simulink model "BH_base_simulink_formigas"  (R2021b)
settings: Solver=ode23tb  StartTime=0.0  StopTime=10  RelTol=1e-3
values from neighbouring files (symbols this model uses):
  a = 3.2    [BH_Otim_formigas.m]
  A1 = 1.2566e-3    (= 0.0012566)    [BH_Otim_formigas.m]
  A2 = 8.765e-4    (= 0.0008765)    [BH_Otim_formigas.m]
  be = 9000e5    (= 900000000)    [BH_Otim_formigas.m]
  f = 1500    [BH_Otim_formigas.m]
  g = 9.8    [BH_Otim_formigas.m]
  gama = 170    [BH_Otim_formigas.m]    (also in cost_func_bh.m = parameter(4))
  k1 = 11    [BH_Otim_formigas.m]    (also in cost_func_bh.m = parameter(5))
  k2 = 0.9    [BH_Otim_formigas.m]    (also in cost_func_bh.m = parameter(6))
  kc1 = 3.644e-12    [BH_Otim_formigas.m]
  kc2 = 4.376e-12    [BH_Otim_formigas.m]
  kq1 = 4.76e-4    (= 0.000476)    [BH_Otim_formigas.m]
  kq2 = 4.76e-4    (= 0.000476)    [BH_Otim_formigas.m]
  M = 84    [BH_Otim_formigas.m]    (also in cost_func_bh.m = M0 + exp(-5*s))
  M0 = 480    [BH_Otim_formigas.m]    (also in cost_func_bh.m = parameter(1))
  r0 = 0.62    [BH_Otim_formigas.m]    (also in cost_func_bh.m = parameter(3))
  V1 = VL1+(A1*xe0)    (= 0.0001330412)    [BH_Otim_formigas.m]
  V2 = VL2+A2*(L-xe0)    (= 0.000153427)    [BH_Otim_formigas.m]
libraries: simulink x1
settings Model: Creator=cof_2  LastModifiedBy=cof_2

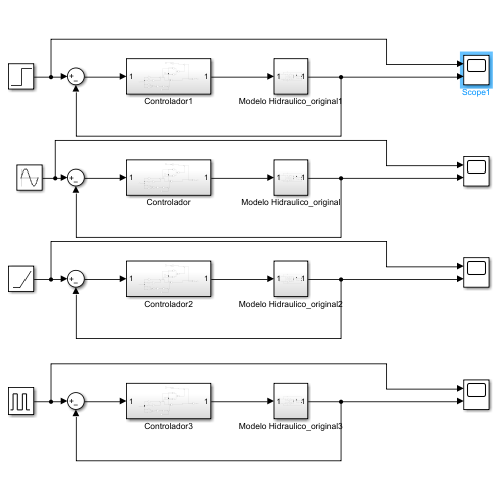
[thumbnail: Simulink's stored preview of the top-level diagram]
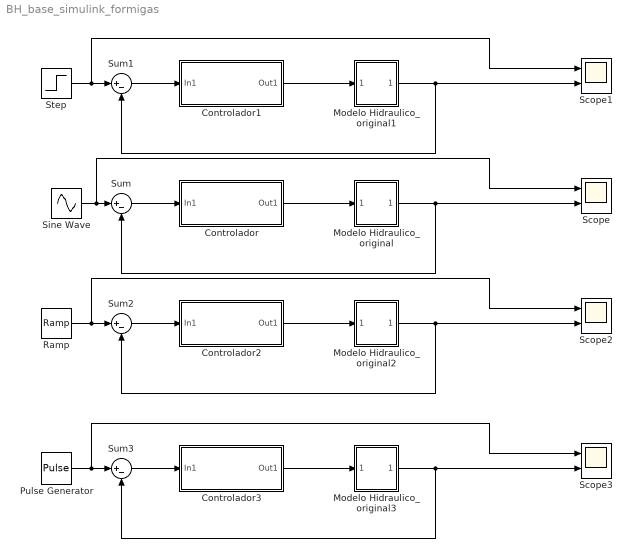
== system BH_base_simulink_formigas ==
  Controlador : Subsystem
  Controlador1 : Subsystem
  Controlador2 : Subsystem
  Controlador3 : Subsystem
  Modelo Hidraulico_original : Subsystem
  Modelo Hidraulico_original1 : Subsystem
  Modelo Hidraulico_original2 : Subsystem
  Modelo Hidraulico_original3 : Subsystem
  Pulse Generator : DiscretePulseGenerator  PulseType=Time based  Period=2.5  PulseWidth=5
  Ramp : simulink/Sources/Ramp  slope=1  start=0  InitialOutput=0
  Scope{,1..3} (4 alike) : Scope  NumInputPorts=2
  Sine Wave : Sin  SampleTime=0
  Step : Step  SampleTime=0
  Sum{,1..3} (4 alike) : Sum  Inputs=|+-
  wires:
  Controlador/1(Out1) -> Modelo Hidraulico_original/1(In1)
  Modelo Hidraulico_original/1(Out1) -> Sum/2, Scope/2
  Sum/1 -> Controlador/1(In1)
  Sine Wave/1 -> Scope/1, Sum/1
  Step/1 -> Sum1/1, Scope1/1
  Sum1/1 -> Controlador1/1(In1)
  Modelo Hidraulico_original1/1(Out1) -> Scope1/2, Sum1/2
  Controlador1/1(Out1) -> Modelo Hidraulico_original1/1(In1)
  Controlador2/1(Out1) -> Modelo Hidraulico_original2/1(In1)
  Modelo Hidraulico_original2/1(Out1) -> Sum2/2, Scope2/2
  Sum2/1 -> Controlador2/1(In1)
  Ramp/1 -> Scope2/1, Sum2/1
  Pulse Generator/1 -> Sum3/1, Scope3/1
  Sum3/1 -> Controlador3/1(In1)
  Modelo Hidraulico_original3/1(Out1) -> Scope3/2, Sum3/2
  Controlador3/1(Out1) -> Modelo Hidraulico_original3/1(In1)

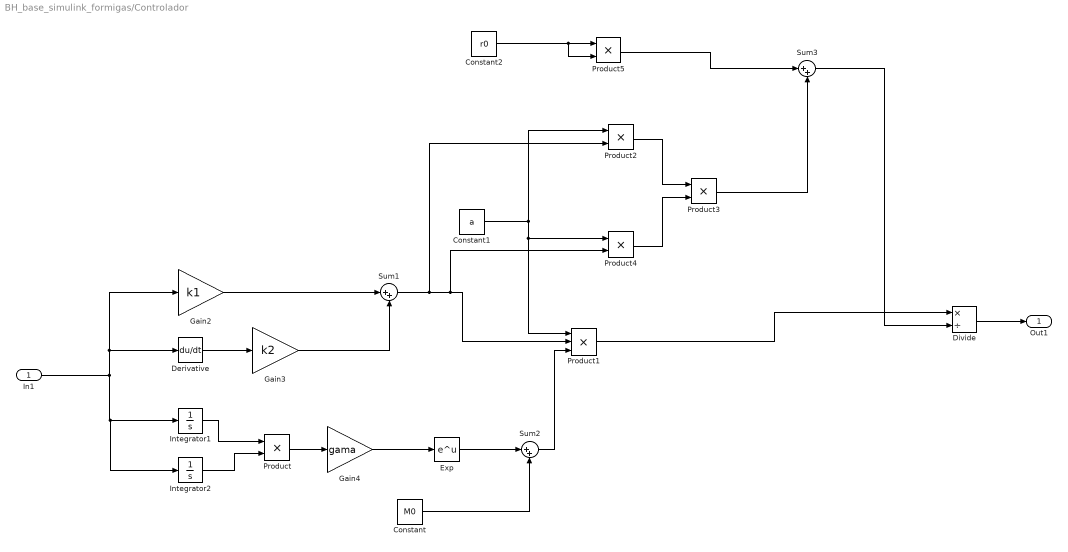
== system BH_base_simulink_formigas/Controlador ==
  In1 : Inport
  Constant : Constant  Value=M0
  Constant1 : Constant  Value=a
  Constant2 : Constant  Value=r0
  Derivative : Derivative
  Divide : Product  Inputs=*/
  Exp : Math  SaturateOnIntegerOverflow=on
  Gain2 : Gain  Gain=k1
  Gain3 : Gain  Gain=k2
  Gain4 : Gain  Gain=gama
  Integrator1 : Integrator
  Integrator2 : Integrator
  Product{,2..5} (5 alike) : Product
  Product1 : Product  Inputs=3
  Sum1 : Sum  Inputs=|++
  Sum2 : Sum  Inputs=|++
  Sum3 : Sum  Inputs=|++
  Out1 : Outport
  wires:
  In1/1 -> Gain2/1, Derivative/1, Integrator2/1, Integrator1/1
  Derivative/1 -> Gain3/1
  Integrator2/1 -> Product/2
  Integrator1/1 -> Product/1
  Product/1 -> Gain4/1
  Gain4/1 -> Exp/1
  Exp/1 -> Sum2/1
  Constant/1 -> Sum2/2
  Gain2/1 -> Sum1/1
  Gain3/1 -> Sum1/2
  Constant1/1 -> Product1/1, Product4/1, Product2/1
  Sum1/1 -> Product2/2, Product4/2, Product1/2
  Sum2/1 -> Product1/3
  Product2/1 -> Product3/1
  Product4/1 -> Product3/2
  Constant2/1 -> Product5/2, Product5/1
  Product5/1 -> Sum3/1
  Product3/1 -> Sum3/2
  Divide/1 -> Out1/1
  Product1/1 -> Divide/1
  Sum3/1 -> Divide/2

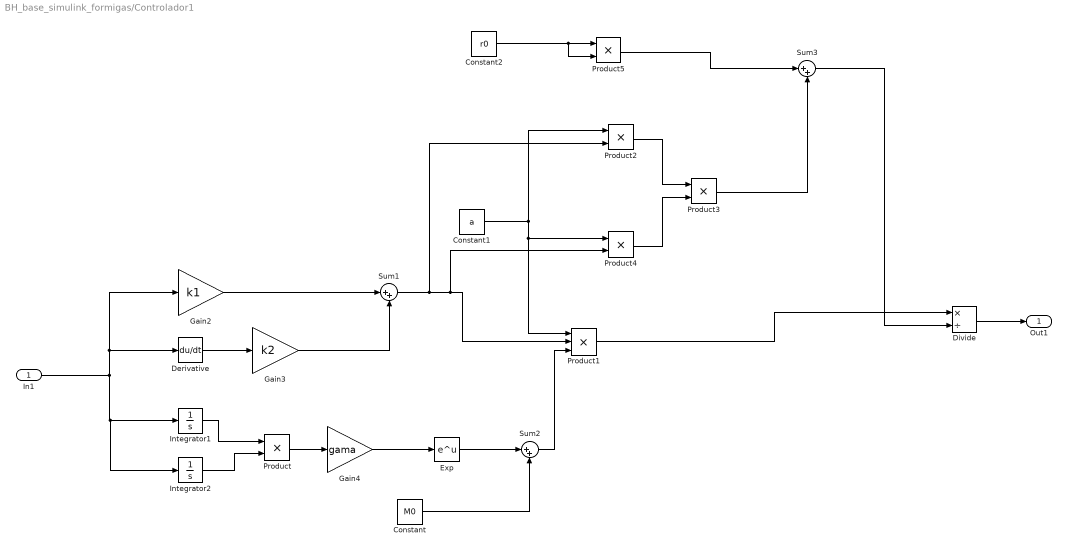
== system BH_base_simulink_formigas/Controlador1 ==
  In1 : Inport
  Constant : Constant  Value=M0
  Constant1 : Constant  Value=a
  Constant2 : Constant  Value=r0
  Derivative : Derivative
  Divide : Product  Inputs=*/
  Exp : Math  SaturateOnIntegerOverflow=on
  Gain2 : Gain  Gain=k1
  Gain3 : Gain  Gain=k2
  Gain4 : Gain  Gain=gama
  Integrator1 : Integrator
  Integrator2 : Integrator
  Product{,2..5} (5 alike) : Product
  Product1 : Product  Inputs=3
  Sum1 : Sum  Inputs=|++
  Sum2 : Sum  Inputs=|++
  Sum3 : Sum  Inputs=|++
  Out1 : Outport
  wires:
  Sum3/1 -> Divide/2
  Product1/1 -> Divide/1
  Divide/1 -> Out1/1
  Product3/1 -> Sum3/2
  Product5/1 -> Sum3/1
  Constant2/1 -> Product5/1, Product5/2
  Product4/1 -> Product3/2
  Product2/1 -> Product3/1
  Sum2/1 -> Product1/3
  Sum1/1 -> Product1/2, Product4/2, Product2/2
  Constant1/1 -> Product2/1, Product4/1, Product1/1
  Gain3/1 -> Sum1/2
  Gain2/1 -> Sum1/1
  Constant/1 -> Sum2/2
  Exp/1 -> Sum2/1
  Gain4/1 -> Exp/1
  Product/1 -> Gain4/1
  Integrator1/1 -> Product/1
  Integrator2/1 -> Product/2
  Derivative/1 -> Gain3/1
  In1/1 -> Integrator1/1, Integrator2/1, Derivative/1, Gain2/1

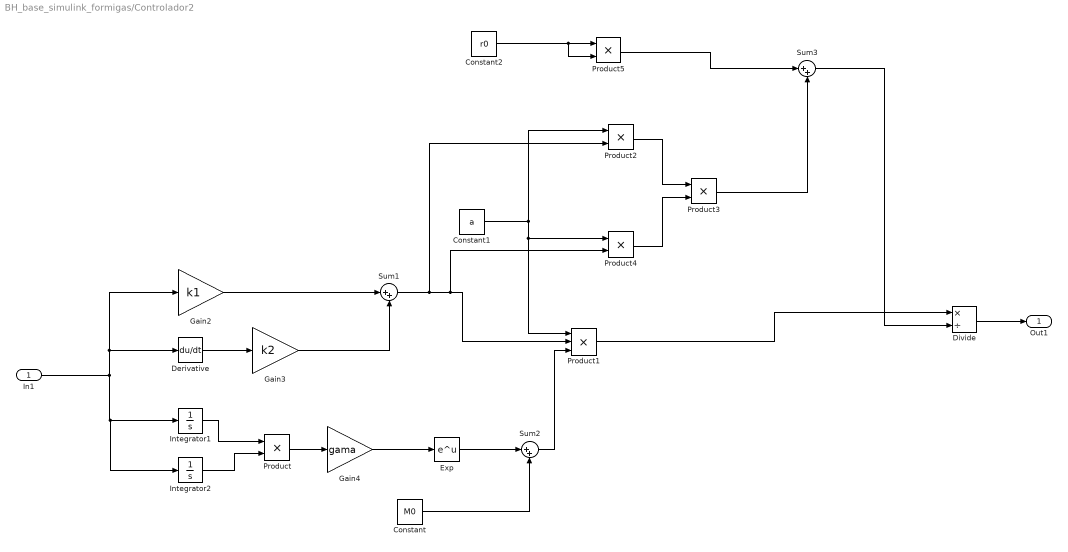
== system BH_base_simulink_formigas/Controlador2 ==
  In1 : Inport
  Constant : Constant  Value=M0
  Constant1 : Constant  Value=a
  Constant2 : Constant  Value=r0
  Derivative : Derivative
  Divide : Product  Inputs=*/
  Exp : Math  SaturateOnIntegerOverflow=on
  Gain2 : Gain  Gain=k1
  Gain3 : Gain  Gain=k2
  Gain4 : Gain  Gain=gama
  Integrator1 : Integrator
  Integrator2 : Integrator
  Product{,2..5} (5 alike) : Product
  Product1 : Product  Inputs=3
  Sum1 : Sum  Inputs=|++
  Sum2 : Sum  Inputs=|++
  Sum3 : Sum  Inputs=|++
  Out1 : Outport
  wires:
  In1/1 -> Gain2/1, Derivative/1, Integrator2/1, Integrator1/1
  Derivative/1 -> Gain3/1
  Integrator2/1 -> Product/2
  Integrator1/1 -> Product/1
  Product/1 -> Gain4/1
  Gain4/1 -> Exp/1
  Exp/1 -> Sum2/1
  Constant/1 -> Sum2/2
  Gain2/1 -> Sum1/1
  Gain3/1 -> Sum1/2
  Constant1/1 -> Product1/1, Product4/1, Product2/1
  Sum1/1 -> Product2/2, Product4/2, Product1/2
  Sum2/1 -> Product1/3
  Product2/1 -> Product3/1
  Product4/1 -> Product3/2
  Constant2/1 -> Product5/2, Product5/1
  Product5/1 -> Sum3/1
  Product3/1 -> Sum3/2
  Divide/1 -> Out1/1
  Product1/1 -> Divide/1
  Sum3/1 -> Divide/2

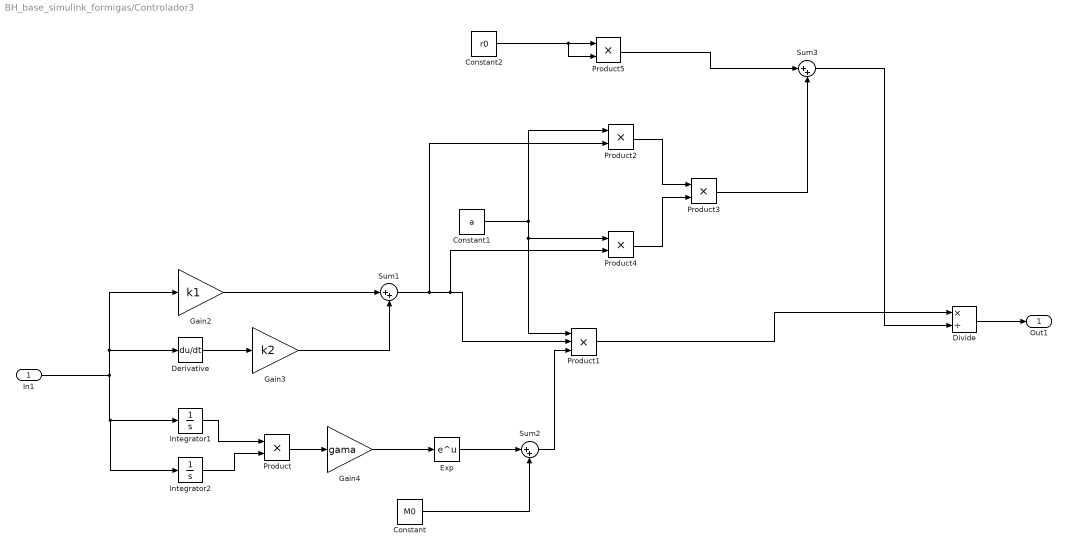
== system BH_base_simulink_formigas/Controlador3 ==
  In1 : Inport
  Constant : Constant  Value=M0
  Constant1 : Constant  Value=a
  Constant2 : Constant  Value=r0
  Derivative : Derivative
  Divide : Product  Inputs=*/
  Exp : Math  SaturateOnIntegerOverflow=on
  Gain2 : Gain  Gain=k1
  Gain3 : Gain  Gain=k2
  Gain4 : Gain  Gain=gama
  Integrator1 : Integrator
  Integrator2 : Integrator
  Product{,2..5} (5 alike) : Product
  Product1 : Product  Inputs=3
  Sum1 : Sum  Inputs=|++
  Sum2 : Sum  Inputs=|++
  Sum3 : Sum  Inputs=|++
  Out1 : Outport
  wires:
  Sum3/1 -> Divide/2
  Product1/1 -> Divide/1
  Divide/1 -> Out1/1
  Product3/1 -> Sum3/2
  Product5/1 -> Sum3/1
  Constant2/1 -> Product5/1, Product5/2
  Product4/1 -> Product3/2
  Product2/1 -> Product3/1
  Sum2/1 -> Product1/3
  Sum1/1 -> Product1/2, Product4/2, Product2/2
  Constant1/1 -> Product2/1, Product4/1, Product1/1
  Gain3/1 -> Sum1/2
  Gain2/1 -> Sum1/1
  Constant/1 -> Sum2/2
  Exp/1 -> Sum2/1
  Gain4/1 -> Exp/1
  Product/1 -> Gain4/1
  Integrator1/1 -> Product/1
  Integrator2/1 -> Product/2
  Derivative/1 -> Gain3/1
  In1/1 -> Integrator1/1, Integrator2/1, Derivative/1, Gain2/1

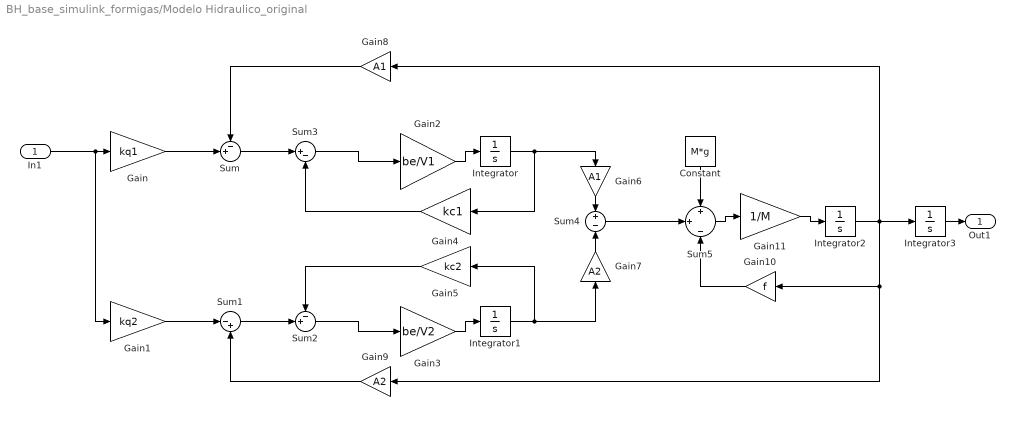
== system BH_base_simulink_formigas/Modelo Hidraulico_original ==
  In1 : Inport
  Constant : Constant  Value=M*g
  Gain : Gain  Gain=kq1
  Gain1 : Gain  Gain=kq2
  Gain10 : Gain  Gain=f
  Gain11 : Gain  Gain=1/M
  Gain2 : Gain  Gain=be/V1
  Gain3 : Gain  Gain=be/V2
  Gain4 : Gain  Gain=kc1
  Gain5 : Gain  Gain=kc2
  Gain6 : Gain  Gain=A1
  Gain7 : Gain  Gain=A2
  Gain8 : Gain  Gain=A1
  Gain9 : Gain  Gain=A2
  Integrator{,1..3} (4 alike) : Integrator
  Sum : Sum  Inputs=-+|
  Sum1 : Sum  Inputs=|-+
  Sum2 : Sum  Inputs=-+|
  Sum3 : Sum  Inputs=|+-
  Sum4 : Sum  Inputs=+|-
  Sum5 : Sum  Inputs=+|+|-
  Out1 : Outport
  wires:
  Sum/1 -> Sum3/1
  Constant/1 -> Sum5/1
  Sum4/1 -> Sum5/2
  Gain6/1 -> Sum4/1
  Integrator1/1 -> Gain7/1, Gain5/1
  Gain1/1 -> Sum1/1
  Integrator/1 -> Gain6/1, Gain4/1
  Sum1/1 -> Sum2/2
  Gain2/1 -> Integrator/1
  Sum5/1 -> Gain11/1
  Gain7/1 -> Sum4/2
  Gain/1 -> Sum/2
  Gain8/1 -> Sum/1
  Sum3/1 -> Gain2/1
  Integrator2/1 -> Gain8/1, Integrator3/1, Gain9/1, Gain10/1
  Gain10/1 -> Sum5/3
  Sum2/1 -> Gain3/1
  Gain5/1 -> Sum2/1
  Gain4/1 -> Sum3/2
  Gain3/1 -> Integrator1/1
  Gain9/1 -> Sum1/2
  Gain11/1 -> Integrator2/1
  In1/1 -> Gain1/1, Gain/1
  Integrator3/1 -> Out1/1

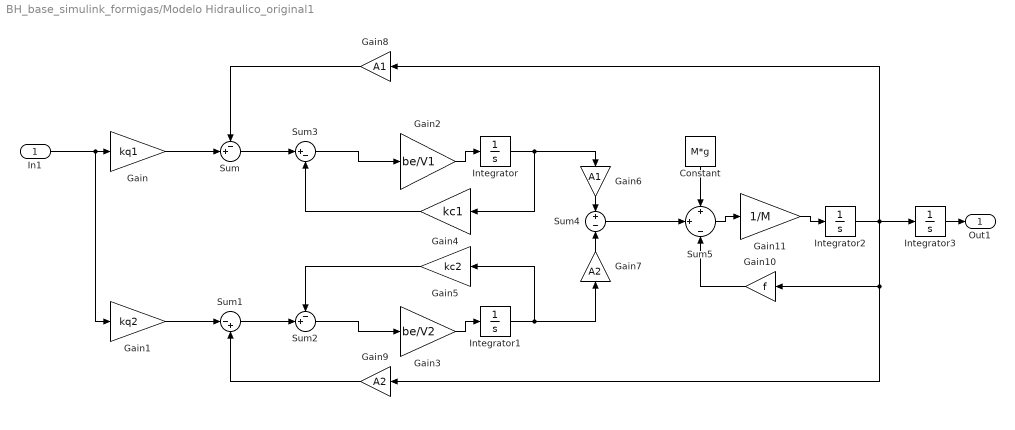
== system BH_base_simulink_formigas/Modelo Hidraulico_original1 ==
  In1 : Inport
  Constant : Constant  Value=M*g
  Gain : Gain  Gain=kq1
  Gain1 : Gain  Gain=kq2
  Gain10 : Gain  Gain=f
  Gain11 : Gain  Gain=1/M
  Gain2 : Gain  Gain=be/V1
  Gain3 : Gain  Gain=be/V2
  Gain4 : Gain  Gain=kc1
  Gain5 : Gain  Gain=kc2
  Gain6 : Gain  Gain=A1
  Gain7 : Gain  Gain=A2
  Gain8 : Gain  Gain=A1
  Gain9 : Gain  Gain=A2
  Integrator{,1..3} (4 alike) : Integrator
  Sum : Sum  Inputs=-+|
  Sum1 : Sum  Inputs=|-+
  Sum2 : Sum  Inputs=-+|
  Sum3 : Sum  Inputs=|+-
  Sum4 : Sum  Inputs=+|-
  Sum5 : Sum  Inputs=+|+|-
  Out1 : Outport
  wires:
  Integrator3/1 -> Out1/1
  In1/1 -> Gain/1, Gain1/1
  Gain11/1 -> Integrator2/1
  Gain9/1 -> Sum1/2
  Gain3/1 -> Integrator1/1
  Gain4/1 -> Sum3/2
  Gain5/1 -> Sum2/1
  Sum2/1 -> Gain3/1
  Gain10/1 -> Sum5/3
  Integrator2/1 -> Gain10/1, Gain9/1, Integrator3/1, Gain8/1
  Sum3/1 -> Gain2/1
  Gain8/1 -> Sum/1
  Gain/1 -> Sum/2
  Gain7/1 -> Sum4/2
  Sum5/1 -> Gain11/1
  Gain2/1 -> Integrator/1
  Sum1/1 -> Sum2/2
  Integrator/1 -> Gain4/1, Gain6/1
  Gain1/1 -> Sum1/1
  Integrator1/1 -> Gain5/1, Gain7/1
  Gain6/1 -> Sum4/1
  Sum4/1 -> Sum5/2
  Constant/1 -> Sum5/1
  Sum/1 -> Sum3/1

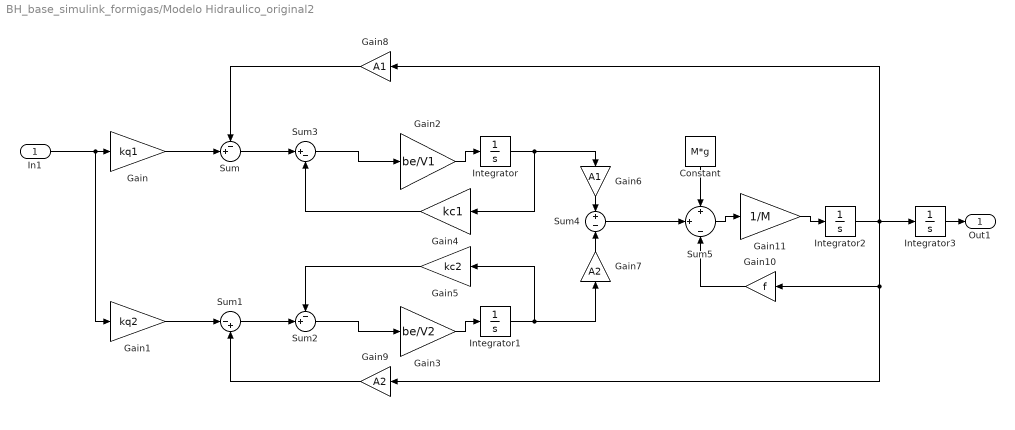
== system BH_base_simulink_formigas/Modelo Hidraulico_original2 ==
  In1 : Inport
  Constant : Constant  Value=M*g
  Gain : Gain  Gain=kq1
  Gain1 : Gain  Gain=kq2
  Gain10 : Gain  Gain=f
  Gain11 : Gain  Gain=1/M
  Gain2 : Gain  Gain=be/V1
  Gain3 : Gain  Gain=be/V2
  Gain4 : Gain  Gain=kc1
  Gain5 : Gain  Gain=kc2
  Gain6 : Gain  Gain=A1
  Gain7 : Gain  Gain=A2
  Gain8 : Gain  Gain=A1
  Gain9 : Gain  Gain=A2
  Integrator{,1..3} (4 alike) : Integrator
  Sum : Sum  Inputs=-+|
  Sum1 : Sum  Inputs=|-+
  Sum2 : Sum  Inputs=-+|
  Sum3 : Sum  Inputs=|+-
  Sum4 : Sum  Inputs=+|-
  Sum5 : Sum  Inputs=+|+|-
  Out1 : Outport
  wires:
  Sum/1 -> Sum3/1
  Constant/1 -> Sum5/1
  Sum4/1 -> Sum5/2
  Gain6/1 -> Sum4/1
  Integrator1/1 -> Gain7/1, Gain5/1
  Gain1/1 -> Sum1/1
  Integrator/1 -> Gain6/1, Gain4/1
  Sum1/1 -> Sum2/2
  Gain2/1 -> Integrator/1
  Sum5/1 -> Gain11/1
  Gain7/1 -> Sum4/2
  Gain/1 -> Sum/2
  Gain8/1 -> Sum/1
  Sum3/1 -> Gain2/1
  Integrator2/1 -> Gain8/1, Integrator3/1, Gain9/1, Gain10/1
  Gain10/1 -> Sum5/3
  Sum2/1 -> Gain3/1
  Gain5/1 -> Sum2/1
  Gain4/1 -> Sum3/2
  Gain3/1 -> Integrator1/1
  Gain9/1 -> Sum1/2
  Gain11/1 -> Integrator2/1
  In1/1 -> Gain1/1, Gain/1
  Integrator3/1 -> Out1/1

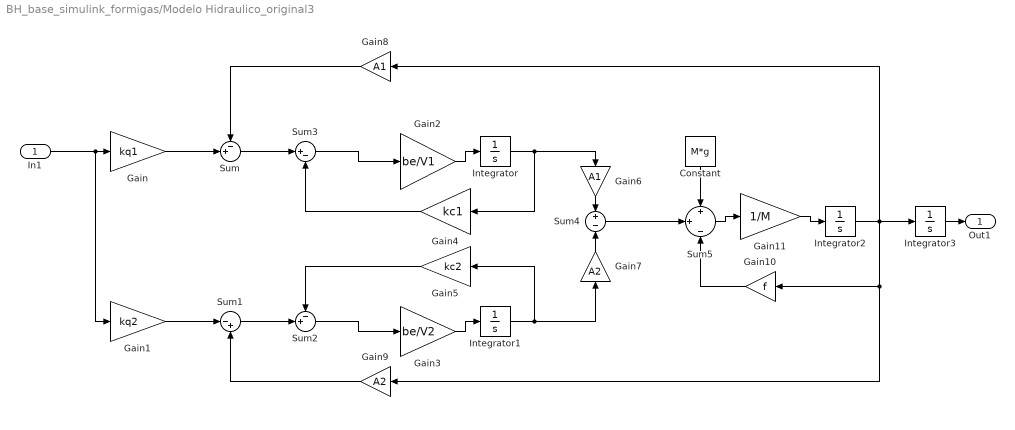
== system BH_base_simulink_formigas/Modelo Hidraulico_original3 ==
  In1 : Inport
  Constant : Constant  Value=M*g
  Gain : Gain  Gain=kq1
  Gain1 : Gain  Gain=kq2
  Gain10 : Gain  Gain=f
  Gain11 : Gain  Gain=1/M
  Gain2 : Gain  Gain=be/V1
  Gain3 : Gain  Gain=be/V2
  Gain4 : Gain  Gain=kc1
  Gain5 : Gain  Gain=kc2
  Gain6 : Gain  Gain=A1
  Gain7 : Gain  Gain=A2
  Gain8 : Gain  Gain=A1
  Gain9 : Gain  Gain=A2
  Integrator{,1..3} (4 alike) : Integrator
  Sum : Sum  Inputs=-+|
  Sum1 : Sum  Inputs=|-+
  Sum2 : Sum  Inputs=-+|
  Sum3 : Sum  Inputs=|+-
  Sum4 : Sum  Inputs=+|-
  Sum5 : Sum  Inputs=+|+|-
  Out1 : Outport
  wires:
  Integrator3/1 -> Out1/1
  In1/1 -> Gain/1, Gain1/1
  Gain11/1 -> Integrator2/1
  Gain9/1 -> Sum1/2
  Gain3/1 -> Integrator1/1
  Gain4/1 -> Sum3/2
  Gain5/1 -> Sum2/1
  Sum2/1 -> Gain3/1
  Gain10/1 -> Sum5/3
  Integrator2/1 -> Gain10/1, Gain9/1, Integrator3/1, Gain8/1
  Sum3/1 -> Gain2/1
  Gain8/1 -> Sum/1
  Gain/1 -> Sum/2
  Gain7/1 -> Sum4/2
  Sum5/1 -> Gain11/1
  Gain2/1 -> Integrator/1
  Sum1/1 -> Sum2/2
  Integrator/1 -> Gain4/1, Gain6/1
  Gain1/1 -> Sum1/1
  Integrator1/1 -> Gain5/1, Gain7/1
  Gain6/1 -> Sum4/1
  Sum4/1 -> Sum5/2
  Constant/1 -> Sum5/1
  Sum/1 -> Sum3/1
